simulink model "ModeloControlePorPressaoRevFinal_Validacao"  (R2017a)
settings: Solver=ode3  StartTime=0.0  StopTime=Tsimulacao  FixedStep=Tamostra  RelTol=1e-3  EnableMultiTasking=on
values from neighbouring files (symbols this model uses):
  Delay = 0.5    [CodigoTeste.m]    (also in Simulacao.m; TesteSimulacao.m; TesteValidacao.m = 0)
  E = 38.1970    (= 38.197)    [CodigoTeste.m]    (also in Simulacao.m; TesteSimulacao.m; TesteValidacao.m)
  PaspMax = Pasp(1,3)    [CodigoTeste.m]    (also in Simulacao.m = Pasp(7,3); TesteSimulacao.m)
  PaspMed = Pasp(1,2)    [CodigoTeste.m]    (also in Simulacao.m = Pasp(7,2); TesteSimulacao.m)
  PaspMin = Pasp(1,1)    [CodigoTeste.m]    (also in Simulacao.m = Pasp(7,1); TesteSimulacao.m)
  PressaoDelay = Pvent    (= 4.6372)    [CodigoTeste.m]    (also in Simulacao.m = Pvent; TesteSimulacao.m = Pvent; TesteValidacao.m = 0)
  Ptrigger = 0.5    [CodigoTeste.m]    (also in Simulacao.m; TesteSimulacao.m; TesteValidacao.m = 0)
  Pvent = 4.6372    [CodigoTeste.m]    (also in Simulacao.m = 5+Indice_PEEP*5; TesteSimulacao.m = 5+Indice_PEEP*5; TesteValidacao.m = 0)
  Rrs = 3.3464    [CodigoTeste.m]    (also in Simulacao.m; TesteSimulacao.m; TesteValidacao.m)
  Tamanho_Sonda = 10    [CodigoTeste.m]    (also in Simulacao.m = 12; TesteSimulacao.m = 6; TesteValidacao.m = str2num(Name(2:3)))
  TOT = 7.5    [CodigoTeste.m]    (also in Simulacao.m = 8.5; TesteResistencias.m = '8.5'; TesteSimulacao.m; TesteValidacao.m = str2num(Name(13:15)))
  VolumeInicial = VR+PressaoInicial/E    (= 0.121402204362)    [CodigoTeste.m]    (also in Simulacao.m = VR+PressaoInicial/E; TesteSimulacao.m = VR+PressaoInicial/E; TesteValidacao.m = 0)
  VR = 0    [CodigoTeste.m]    (also in Simulacao.m; TesteSimulacao.m; TesteValidacao.m)
libraries: simulink x1
settings Model: Creator=Proprietário  LastModifiedBy=Texugão
settings DataIOCC: LimitDataPoints=on  SaveFormat=Array
settings OptimizationCC: LifeSpan=inf
settings DebuggingCC: SolverPrmCheckMsg=warning  SFUnexpectedBacktrackingDiag=warning  SFNoUnconditionalDefaultTransitionDiag=warning  SFExecutionAtInitializationDiag=none
settings HardwareCC: ProdBitPerPointer=32  ProdBitPerSizeT=32  ProdBitPerPtrDiffT=32  ProdLargestAtomicFloat=None  ProdIntDivRoundTo=Undefined  ProdEndianess=Unspecified  ProdWordSize=32  ProdHWDeviceType=32-bit Generic
settings ModelReferenceCC: PropagateSignalLabelsOutOfModel=off
settings GRTTargetCC: TargetLangStandard=C89/C90 (ANSI)  GeneratePreprocessorConditionals=Disable all
settings ConfigComp: CovMetricSettings=dw  CovHtmlReporting=on  CovSaveCumulativeToWorkspaceVar=on  CovSaveSingleToWorkspaceVar=on  CovExternalEMLEnable=off  CovSFcnEnable=off

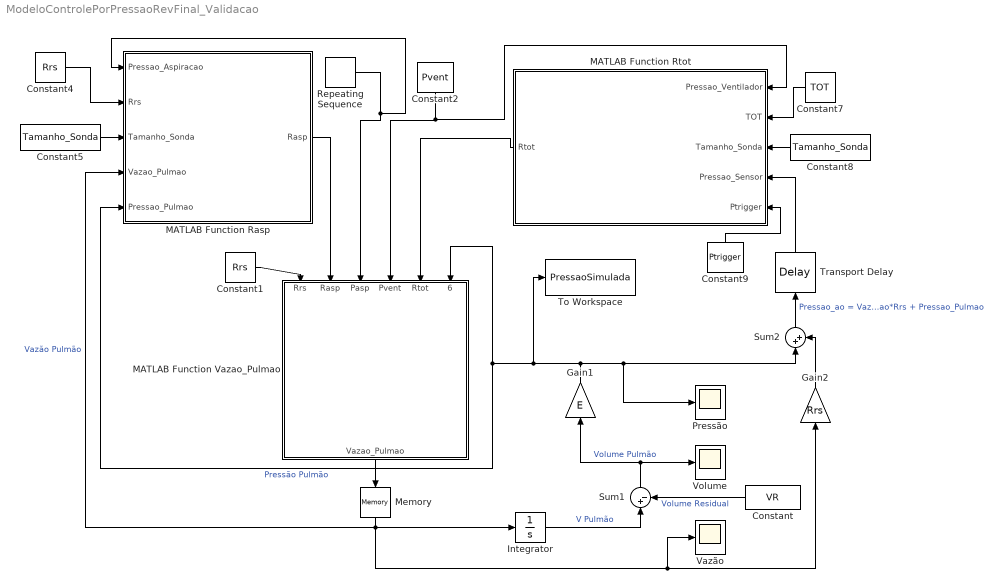
== system ModeloControlePorPressaoRevFinal_Validacao ==
  Constant : Constant  Value=VR
  Constant1 : Constant  Value=Rrs
  Constant2 : Constant  Value=Pvent
  Constant4 : Constant  Value=Rrs
  Constant5 : Constant  Value=Tamanho_Sonda
  Constant7 : Constant  Value=TOT
  Constant8 : Constant  Value=Tamanho_Sonda
  Constant9 : Constant  Value=Ptrigger
  Gain1 : Gain  Gain=E
  Gain2 : Gain  Gain=Rrs
  Integrator : Integrator  InitialCondition=VolumeInicial
  MATLAB Function Rasp : MATLAB Function  TreatAsAtomicUnit=on
  MATLAB Function Rtot : MATLAB Function  TreatAsAtomicUnit=on
  MATLAB Function Vazao_Pulmao : MATLAB Function  TreatAsAtomicUnit=on
  Memory : Memory
  Pressão : Scope
  Repeating Sequence : simulink/Sources/Repeating Sequence  rep_seq_t=[0 5 5+0.001 20 20+0.001 40 40+0.001 55 55+0.001 75 75+0.001 90 90+0.001 95]  rep_seq_y=[0 0 PaspMin PaspMin 0 0 PaspMed PaspMed 0 0 PaspMax PaspMax 0 0]
  Sum1 : Sum  Inputs=|+-
  Sum2 : Sum  Inputs=|++
  To Workspace : ToWorkspace  VariableName=PressaoSimulada  SaveFormat=Timeseries  SampleTime=-1
  Transport Delay : TransportDelay  DelayTime=Delay  InitialOutput=PressaoDelay
  Vazão : Scope
  Volume : Scope
  wires:
  Integrator/1 -> Sum1/1  "V Pulmão"
  Constant/1 -> Sum1/2  "Volume Residual"
  Memory/1 -> Vazão/1, Gain2/1, MATLAB Function Rasp/4(Vazao_Pulmao), Integrator/1  "Vazão Pulmão"
  Sum1/1 -> Gain1/1, Volume/1  "Volume Pulmão"
  Gain1/1 -> Sum2/1, Pressão/1, To Workspace/1, MATLAB Function Rasp/5(Pressao_Pulmao), MATLAB Function Vazao_Pulmao/6(Pressao_Pulmao)  "Pressão Pulmão"
  MATLAB Function Rasp/1(Rasp) -> MATLAB Function Vazao_Pulmao/2(Rasp)
  MATLAB Function Rtot/1(Rtot) -> MATLAB Function Vazao_Pulmao/5(Rtot)
  Constant2/1 -> MATLAB Function Rtot/1(Pressao_Ventilador), MATLAB Function Vazao_Pulmao/4(Pvent)
  MATLAB Function Vazao_Pulmao/1(Vazao_Pulmao) -> Memory/1
  Constant4/1 -> MATLAB Function Rasp/2(Rrs)
  Constant5/1 -> MATLAB Function Rasp/3(Tamanho_Sonda)
  Constant8/1 -> MATLAB Function Rtot/3(Tamanho_Sonda)
  Constant7/1 -> MATLAB Function Rtot/2(TOT)
  Constant1/1 -> MATLAB Function Vazao_Pulmao/1(Rrs)
  Repeating Sequence/1 -> MATLAB Function Vazao_Pulmao/3(Pasp), MATLAB Function Rasp/1(Pressao_Aspiracao)
  Gain2/1 -> Sum2/2
  Sum2/1 -> Transport Delay/1  "Pressao_ao = Vazao_Pulmao*Rrs + Pressao_Pulmao"
  Transport Delay/1 -> MATLAB Function Rtot/4(Pressao_Sensor)
  Constant9/1 -> MATLAB Function Rtot/5(Ptrigger)

== matlab function ModeloControlePorPressaoRevFinal_Validacao/MATLAB Function Rasp ==
  data: Pressao_Aspiracao input; Rrs input; Tamanho_Sonda input; Vazao_Pulmao input; Rasp output; Pressao_Pulmao input
function Rasp  = Resistencia_da_Sonda_de_Aspiracao(Pressao_Aspiracao, Rrs, Tamanho_Sonda, Vazao_Pulmao, Pressao_Pulmao)

%Equação de movimento para o sistema respiratório
Pressao_ao = Vazao_Pulmao*Rrs + Pressao_Pulmao; 

Delta_P = abs(Pressao_Aspiracao - Pressao_ao);

%Estimação da Vazão de acordo com o Tamanho da Sonda utilizada [00, 06, 08, 10, ou 12]
Vazao = 1;
Rasp = 1;
if Tamanho_Sonda == 0
    Vazao = 0;
elseif Tamanho_Sonda == 06
    Vazao = 0.001339*Delta_P^0.7939;   
elseif Tamanho_Sonda == 08
    Vazao = 0.01081*Delta_P^0.6338;
elseif Tamanho_Sonda == 10
    Vazao = 0.01501*Delta_P^0.6046;
elseif Tamanho_Sonda == 12
    Vazao = 0.03048*Delta_P^0.5689;
elseif Tamanho_Sonda == 14
    Vazao = 0.05087*Delta_P^0.5644;
end

%Rasp
if Vazao == 0
    Rasp = 0;
else
    Rasp = Delta_P/Vazao;
end

== matlab function ModeloControlePorPressaoRevFinal_Validacao/MATLAB Function Rtot ==
  data: Pressao_Ventilador input; TOT input; Tamanho_Sonda input; Pressao_Sensor input; Rtot output; Ptrigger input
function Rtot  = Resistencia_do_TOT(Pressao_Ventilador, TOT, Tamanho_Sonda, Pressao_Sensor, Ptrigger)

Delta_P = abs(Pressao_Ventilador - Pressao_Sensor);

%Sensibilidade do Ventilador
persistent Status_Ventilador; %A variável Status_Ventilador mantem o valor entre execuções
if isempty(Status_Ventilador)
    %Se está vazio, começa desligado
    Status_Ventilador=false;
end
if Delta_P == 0     
    %Desliga o Ventilador
    Status_Ventilador = false;
elseif Delta_P > Ptrigger
    %Ativa o ventilador
    Status_Ventilador = true;
end

if Status_Ventilador
    %Mantem o Delta_P
else
    %Se o ventilador desligado, não tem vazão
    Delta_P =0;
end 

%Estimação da Vazão de acordo com a combinação de TOT [7.5 ou 8.5] e Tamanho da Sonda utilizada [00, 06, 08, 10, ou 12]
Vazao = 1;
Rtot = 1;
if TOT == 7.5
    if Tamanho_Sonda == 0
        Vazao = 0.3833*Delta_P^0.5872;
    elseif Tamanho_Sonda == 06
        Vazao = 0.3223*Delta_P^0.5745;
    elseif Tamanho_Sonda == 08
        Vazao = 0.2745*Delta_P^0.5687;
    elseif Tamanho_Sonda == 10
        Vazao = 0.2682*Delta_P^0.5726;
    end
elseif TOT == 8.5
    if Tamanho_Sonda == 0
        Vazao = 0.548*Delta_P^0.5688;
    elseif Tamanho_Sonda == 06
        Vazao = 0.4413*Delta_P^0.5807;
    elseif Tamanho_Sonda == 08
        Vazao = 0.3795*Delta_P^0.5819;
    elseif Tamanho_Sonda == 10
        Vazao = 0.3808*Delta_P^0.5843;
    elseif Tamanho_Sonda == 12
        Vazao = 0.321*Delta_P^0.5871;
    end
end

if Vazao == 0
    Rtot = 0;
elseif Vazao > 0.5 %Vazão máxima do ventilador
    Vazao = 0.5;
    Rtot = Delta_P/Vazao;
else
    Rtot = Delta_P/Vazao;
end

== matlab function ModeloControlePorPressaoRevFinal_Validacao/MATLAB Function Vazao_Pulmao ==
  data: Rrs input; Rasp input; Vazao_Pulmao output; Pasp input; Pvent input; Rtot input; Pressao_Pulmao input
function Vazao_Pulmao = Lei_de_Conservacao_da_Massa(Rrs, Rasp, Pasp, Pvent, Rtot, Pressao_Pulmao)

if Rasp == 0
    if Rtot == 0
        %Sistema em equilibrio -> V' = -E(V-VR)/Rrs
        Vazao_Pulmao = 0;
    else
        %Sem circuito de aspiração -> V' = (Pvent/Rtot -E(V-VR)/Rtot)/(1+(Rrs/Rtot))
        Vazao_Pulmao = (Pvent/Rtot - Pressao_Pulmao*(1/Rtot))/(1+(Rrs/Rtot));
    end
    
elseif Rtot == 0
    %Diferença entre delta_P do Pulmão e Ventilador = 0 -> V' = (Pasp/Rasp -E(V-VR)/Rasp)/(1+(Rrs/Rasp))
    Vazao_Pulmao = (Pasp/Rasp - Pressao_Pulmao*(1/Rasp))/(1+(Rrs/Rasp));
else
    %Funcionamento Normal
    Vazao_Pulmao = (Pasp/Rasp + Pvent/Rtot - Pressao_Pulmao*(1/Rasp+1/Rtot))/(1+(1/Rtot+1/Rasp)*Rrs);
end
